simulink model "LICENTA_2024v8"  (R2018b)
settings: Solver=FixedStepDiscrete  StartTime=0.0  StopTime=Inf  RelTol=1e-3  EnableMultiTasking=on
values from neighbouring files (symbols this model uses):
  factor_conversie = (1/Rshunt)*(1/10)*(vref/4095)    (= 0.0115122972266)    [licentam18.m]
  FED = uint16(50)    [licentam18.m]
  MaxIter_1_ms_eCAP_wait = MinDetectSpeed_period/T_pos    (= 375)    [licentam18.m]
  offset_ADC = xT*4095/vref    (= 2047.5)    [licentam18.m]
  pp = 16/2    (= 8)    [licentam18.m]
  RED = uint16(50)    [licentam18.m]
  T_pos = 5*10^-4    (= 0.0005)    [licentam18.m]
  TBPRD1 = uint16(TPWM/(2*TTBCLK))    [licentam18.m]
  Tf = 0.015    [licentam18.m]
  Tf_spd = 0.01    [licentam18.m]
  TiSamplePos = T_pos    (= 0.0005)    [licentam18.m]
  Ts = Ts_crt_control    (= 3.33333333333e-05)    [licentam18.m]
  TTBCLK = 1/F    (= 5e-09)    [licentam18.m]
undefined symbols (not defined in the file or in its folder): Discrete, Down, GPTRIP1SEL, GPTRIP2SEL, radians, Time, TZ1, TZ2, Up
libraries: tiiqmathlib x25, c2802xlib x6, c2837xDlib x6, c280xlib x4, simulink x3, ctrlSharedLib x2, c2000lib x1, c28xdmclib x1
(part 1 of 2)
settings Model: ExtModeTrigDuration=8  Creator=mocan  LastModifiedBy=antic
settings SolverCC: AutoInsertRateTranBlk=on
settings OptimizationCC: DefaultUnderspecifiedDataType=single  EnhancedBackFolding=on  PassReuseOutputArgsAs=Individual arguments  MaxStackSize=512  OptimizeBlockOrder=speed  DifferentSizesBufferReuse=on  OptimizationCustomize=off
settings DebuggingCC: ParameterPrecisionLossMsg=none  ParameterTunabilityLossMsg=error
settings HardwareCC: ProdBitPerChar=16  ProdBitPerInt=16  ProdBitPerPointer=32  ProdBitPerSizeT=32  ProdBitPerPtrDiffT=32  ProdLargestAtomicInteger=Integer  ProdLargestAtomicFloat=None  ProdWordSize=16  ProdLongLongMode=on  ProdHWDeviceType=Texas Instruments->C2000
settings SFSimCC: MATLABDynamicMemAlloc=off
settings RTWCC: SystemTargetFile=ert.tlc  HardwareBoard=TI Delfino F28379D LaunchPad  TemplateMakefile=ert_default_tmf  GenerateReport=on  Toolchain=Texas Instruments Code Composer Studio (C2000)  IncludeHyperlinkInReport=on  LaunchReport=on  GenerateTraceInfo=on  GenerateTraceReport=on  GenerateTraceReportSl=on  GenerateTraceReportSf=on  GenerateTraceReportEml=on
settings CodeAppCC: ForceParamTrailComments=on  IgnoreCustomStorageClasses=off  OperatorAnnotations=on  SimulinkDataObjDesc=on  SFDataObjDesc=on  InsertBlockDesc=on
settings ERTTargetCC: CodeReplacementLibrary=TI C28x

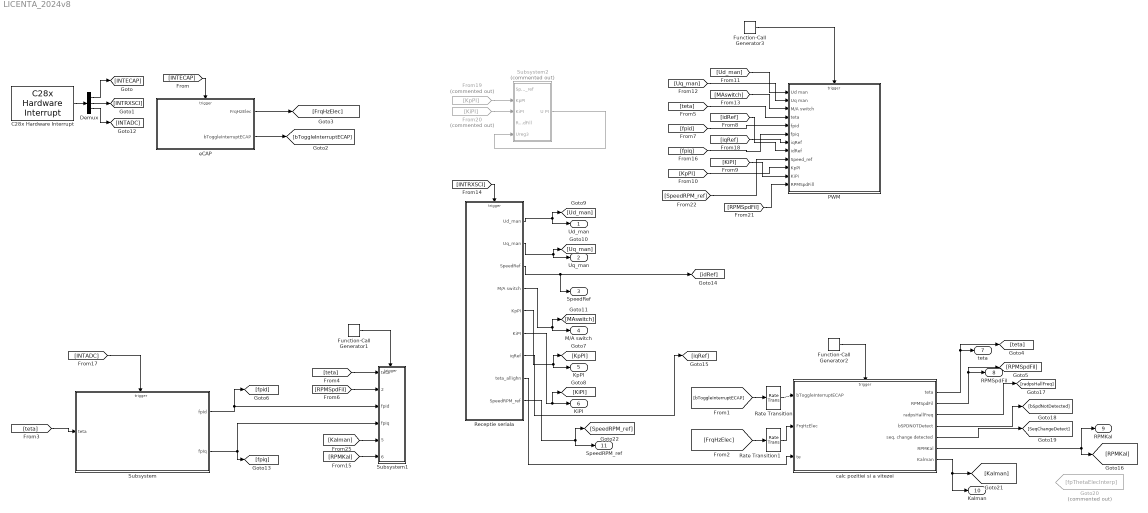
== system LICENTA_2024v8 ==
  C28x Hardware Interrupt : c2000lib/Scheduling/C28x Hardware Interrupt  irqnumbers=[4,9,1]  pienumbers=[1,1,1]  irqpriorities=[1, 1, 1]  irqpreempts=[0 0 0]  showinput=off  dspchiptype=C280X
      settings: SourceProductBaseCode=TIC2000
  Demux : Demux  Outputs=3
  From19 : From  Commented=on  GotoTag=KpPI
  From20 : From  Commented=on  GotoTag=KiPI
  Function-Call Generator1 : simulink/Ports & Subsystems/Function-Call Generator  sample_time=0.03  numberOfIterations=1
  Function-Call Generator2 : simulink/Ports & Subsystems/Function-Call Generator  sample_time=T_pos  numberOfIterations=1
  Function-Call Generator3 : simulink/Ports & Subsystems/Function-Call Generator  sample_time=Ts_crt_control  numberOfIterations=1
  Goto20 : Goto  Commented=on  GotoTag=fpThetaElecInterp
  PWM : Subsystem
  Rate Transition : RateTransition  Integrity=off  OutPortSampleTime=T_pos
  Rate Transition1 : RateTransition  Integrity=off  OutPortSampleTime=T_pos
  "Receptie seriala " : Subsystem
  Subsystem : Subsystem
  Subsystem1 : Subsystem
  Subsystem2 : Subsystem  Commented=on
  calc pozitiei si a vitezei : Subsystem
  eCAP : Subsystem
  Ud_man : Outport  VectorParamsAs1DForOutWhenUnconnected=on
  Uq_man : Outport  Port=2  VectorParamsAs1DForOutWhenUnconnected=on
  SpeedRef : Outport  Port=3  VectorParamsAs1DForOutWhenUnconnected=on
  M/A switch : Outport  Port=4  VectorParamsAs1DForOutWhenUnconnected=on
  KpPI : Outport  Port=5  VectorParamsAs1DForOutWhenUnconnected=on
  KiPI : Outport  Port=6  VectorParamsAs1DForOutWhenUnconnected=on
  teta : Outport  Port=7  VectorParamsAs1DForOutWhenUnconnected=on
  RPMSpdFil : Outport  Port=8  VectorParamsAs1DForOutWhenUnconnected=on
  RPMKal : Outport  Port=9  VectorParamsAs1DForOutWhenUnconnected=on
  Kalman : Outport  Port=10
  SpeedRPM_ref : Outport  Port=11  VectorParamsAs1DForOutWhenUnconnected=on
  wires:
  Rate Transition1/1 -> calc pozitiei si a vitezei/2(FrqHzElec)
  [FrqHzElec] -> Rate Transition1/1
  Rate Transition/1 -> calc pozitiei si a vitezei/1(bToggleInterruptECAP)
  [bToggleInterruptECAP] -> Rate Transition/1
  [INTECAP] -> eCAP/Trigger
  eCAP/1(FrqHzElec) -> [FrqHzElec]
  eCAP/2(bToggleInterruptECAP) -> [bToggleInterruptECAP]
  Demux/2 -> [INTRXSCI]
  Demux/1 -> [INTECAP]
  Function-Call Generator2/1 -> calc pozitiei si a vitezei/Trigger
  calc pozitiei si a vitezei/2(RPMSpdFil) -> [RPMSpdFil], RPMSpdFil/1
  Function-Call Generator1/1 -> Subsystem1/Trigger
  calc pozitiei si a vitezei/1(teta) -> [teta], teta/1
  [INTRXSCI] -> "Receptie seriala "/Trigger
  C28x Hardware Interrupt/1 -> Demux/1
  "Receptie seriala "/1(Ud_man) -> Ud_man/1, [Ud_man]
  "Receptie seriala "/2(Uq_man) -> Uq_man/1, [Uq_man]
  "Receptie seriala "/4(M/A switch) -> M/A switch/1, [MAswitch]
  "Receptie seriala "/5(KpPI) -> KpPI/1, [KpPI]
  "Receptie seriala "/6(KiPI) -> [KiPI], KiPI/1
  Function-Call Generator3/1 -> PWM/Trigger
  Demux/3 -> [INTADC]
  [INTADC] -> Subsystem/Trigger
  [teta] -> Subsystem/1(teta)
  Subsystem/1(fpId) -> [fpid], Subsystem1/3(fpId)
  Subsystem/2(fpIq) -> Subsystem1/4(fpIq), [fpiq]
  "Receptie seriala "/7(iqRef) -> [iqRef]
  "Receptie seriala "/3(SpeedRef) -> SpeedRef/1, [idRef]
  [Ud_man] -> PWM/1(Ud man)
  [Uq_man] -> PWM/2("Uq man ")
  [MAswitch] -> PWM/3(M/A switch)
  [teta] -> PWM/4("teta ")
  [idRef] -> PWM/8(idRef)
  [fpid] -> PWM/5(fpid)
  [fpiq] -> PWM/6(fpiq)
  [iqRef] -> PWM/7("iqRef ")
  [KiPI] -> PWM/11("KiPi ")
  [KpPI] -> PWM/10(KpPI)
  [RPMSpdFil] -> Subsystem1/2("RPMSpdFil ")
  "Receptie seriala "/8(teta_allighn) -> calc pozitiei si a vitezei/3(te)
  calc pozitiei si a vitezei/3(radpsHallFreq) -> [radpsHallFreq]
  calc pozitiei si a vitezei/4("bSPDNOTDetect ") -> [bSpdNotDetected]
  calc pozitiei si a vitezei/5("seq. change detected ") -> [SeqChangeDetect]
  [teta] -> Subsystem1/1("teta ")
  [RPMKal] -> Subsystem1/6(RPMKal)
  calc pozitiei si a vitezei/6(RPMKal) -> RPMKal/1, [RPMKal]
  calc pozitiei si a vitezei/7(Kalman) -> Kalman/1, [Kalman]
  [Kalman] -> Subsystem1/5(Kalman)
  "Receptie seriala "/9("SpeedRPM_ref ") -> [SpeedRPM_ref], SpeedRPM_ref/1
  From20/1 -> Subsystem2/3(KiPI)
  Subsystem2/1("U PI ") -> Subsystem2/5(Ureg3)
  From19/1 -> Subsystem2/2(KpPI)
  [SpeedRPM_ref] -> PWM/9(Speed_ref)
  [RPMSpdFil] -> PWM/12(RPMSpdFill)

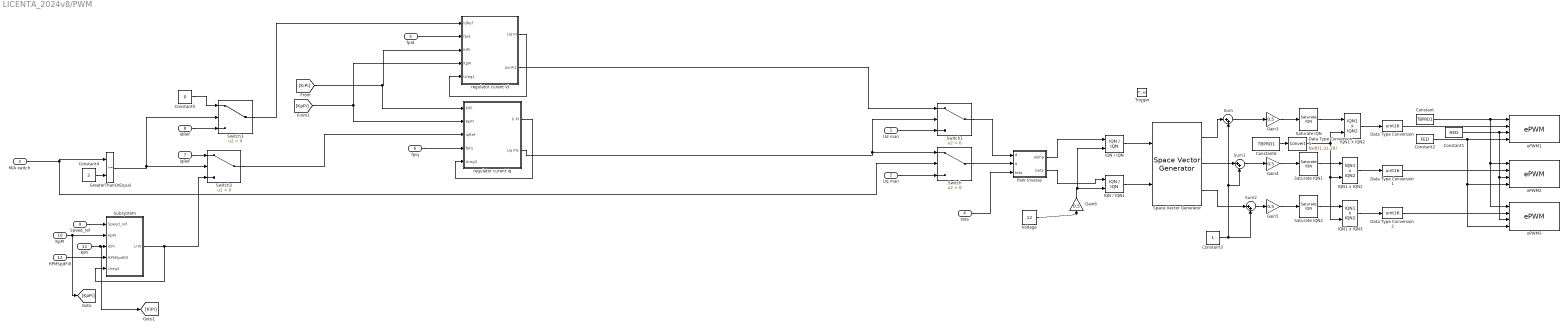
== system LICENTA_2024v8/PWM ==
  Ud man : Inport
  "Uq man " : Inport  Port=2
  M/A switch : Inport  Port=3
  "teta " : Inport  Port=4
  fpid : Inport  Port=5
  fpiq : Inport  Port=6
  "iqRef " : Inport  Port=7
  idRef : Inport  Port=8
  Speed_ref : Inport  Port=9
  KpPI : Inport  Port=10
  "KiPi " : Inport  Port=11
  RPMSpdFill : Inport  Port=12
  Trigger : TriggerPort  TriggerType=function-call  VariantControl=Variant  PortDimensions=1
  Constant : Constant  Value=TBPRD1
  Constant1 : Constant  Value=RED
  Constant2 : Constant  Value=FED
  Constant3 : Constant  OutDataTypeStr=fixdt(1,32,24)
  Constant4 : Constant  Value=2
  Constant5 : Constant  Value=0
  Constant6 : Constant  Value=TBPRD1
  Data Type Conversion : DataTypeConversion  OutDataTypeStr=uint16
  Data Type Conversion1 : DataTypeConversion  OutDataTypeStr=uint16
  Data Type Conversion2 : DataTypeConversion  OutDataTypeStr=uint16
  Data Type Conversion5 : DataTypeConversion  OutDataTypeStr=fixdt(1,32,18)
  Gain{3..6} (4 alike) : Gain  Gain=0.5  OutDataTypeStr=Inherit: Same as input
  GreaterThanOrEqual : RelationalOperator  OutDataTypeStr=boolean  RndMeth=Simplest
  IQN / IQN : tiiqmathlib/IQN // IQN
      settings: SourceProductName=Embedded Coder Support Package for Texas Instruments C2000 Processors  SourceProductBaseCode=TIC2000
  IQN / IQN1 : tiiqmathlib/IQN // IQN
      settings: SourceProductName=Embedded Coder Support Package for Texas Instruments C2000 Processors  SourceProductBaseCode=TIC2000
  IQN1 x IQN1 : tiiqmathlib/IQN1 x IQN2  Q=10
      settings: SourceProductName=Embedded Coder Support Package for Texas Instruments C2000 Processors  SourceProductBaseCode=TIC2000
  IQN1 x IQN2 : tiiqmathlib/IQN1 x IQN2  Q=10
      settings: SourceProductName=Embedded Coder Support Package for Texas Instruments C2000 Processors  SourceProductBaseCode=TIC2000
  IQN1 x IQN3 : tiiqmathlib/IQN1 x IQN2  Q=10
      settings: SourceProductName=Embedded Coder Support Package for Texas Instruments C2000 Processors  SourceProductBaseCode=TIC2000
  Park Inverse : Subsystem
  Saturate IQN : tiiqmathlib/Saturate IQN  pos=0.95  neg=0.05
      settings: SourceProductName=Embedded Coder Support Package for Texas Instruments C2000 Processors  SourceProductBaseCode=TIC2000
  Saturate IQN1 : tiiqmathlib/Saturate IQN  pos=0.95  neg=0.05
      settings: SourceProductName=Embedded Coder Support Package for Texas Instruments C2000 Processors  SourceProductBaseCode=TIC2000
  Saturate IQN2 : tiiqmathlib/Saturate IQN  pos=0.95  neg=0.05
      settings: SourceProductName=Embedded Coder Support Package for Texas Instruments C2000 Processors  SourceProductBaseCode=TIC2000
  Space Vector Generator : c28xdmclib/Space Vector Generator
      settings: SourceProductName=Embedded Coder Support Package for Texas Instruments C2000 Processors  SourceProductBaseCode=TIC2000
  Subsystem : Subsystem
  Sum : Sum  Inputs=|++
  Sum1 : Sum  Inputs=|++
  Sum2 : Sum  Inputs=|++
  Switch{,1..3} (4 alike) : Switch  Criteria=u2 > Threshold
  "Voltage " : Constant  Value=12  OutDataTypeStr=fixdt(1,32,20)
  ePWM1 : c2802xlib/ePWM  useModule=ePWM1  ePWMxLINKTBPRD=Not Linked  periodUnits=Clock cycles  timerSource=Input port  timerPeriod_clk=TBPRD1+1  timerPeriod_sec=0.0001  tbshadow=Counter equals to zero  countingMode=Up-Down  phaseActiveEnable=Disable  phaseDirection=Count up after sync  phaseActive=0  synchronizationEnable=off  dcaevt1Sync=off  dcbevt1Sync=off  synchronizationOption=Counter equals to zero (CTR=Zero)  clockPrescale=1  HSclockPrescale=1  enswap=off  ePWMxAStatus=on  ePWMxAactionLogic1=Do nothing  ePWMxAactionLogic2=Do nothing  ePWMxAactionLogic3=Clear  ePWMxAactionLogic4=Set  ePWMxAactionLogic5=Do nothing  ePWMxAactionLogic6=Do nothing  ePWMxALoadMode=Load on counter equals to zero (CTR=Zero)  ePWMxACSFenable=off  ePWMxACSFvalue=Forcing disable  ePWMxASFreload=Zero  ePWMxBStatus=off  ePWMxBactionLogic1=Set  ePWMxBactionLogic2=Clear  ePWMxBactionLogic3=Do nothing  ePWMxBactionLogic4=Do nothing  ePWMxBactionLogic5=Clear  ePWMxBactionLogic6=Set  ePWMxBLoadMode=Load on counter equals to zero (CTR=Zero)  ePWMxBCSFenable=off  ePWMxBCSFvalue=Forcing disable  ePWMxBSFreload=Zero  ePWNxBOutWay=off  ePWMxLINKCMPA=Not Linked  CMPAUnits=Clock cycles  CMPASource=Input port  CMPAValue_per=50  CMPAValue_clk=0  enCMPAshadow=Counter equals to zero  ePWMxLINKCMPB=Not Linked  CMPBUnits=Clock cycles  CMPBSource=Specify via dialog  CMPBValue_per=50  CMPBValue_clk=0  enCMPBshadow=Counter equals to zero  ePWMxLINKCMPC=Not Linked  CMPCUnits=Clock cycles  CMPCSource=Specify via dialog  CMPCValue_per=50  CMPCValue_clk=32000  enCMPCshadow=Counter equals to zero  ePWMxLINKCMPD=Not Linked  CMPDUnits=Clock cycles  CMPDSource=Specify via dialog  CMPDValue_per=50  CMPDValue_clk=32000  enCMPDshadow=Counter equals to zero  enableDBePWMxA=on  enableDBePWMxB=on  enhalfcycle=off  DBpolarity=Active high complementary (AHC)  DBedgeDelay=Positive  DBSource_ePWMxA=ePWMxA  DBSource_ePWMxB=ePWMxA  DBperiodSource=Input port  REDperiod=0  FEDperiod=0  adcstartModuleA=on  adcrequestEventA=First event  adcstartEventA=Digital Compare Module A Event 1 start of conversion (DCAEVT1.soc)  adcstartEventA_type2=Counter equals to period (CTR=PRD)  adcstartModuleB=off  adcrequestEventB=First event  adcstartEventB=Counter equals to zero (CTR=Zero)  adcstartEventB_type2=Counter equals to zero (CTR=Zero)  intEn=off  intPrd=First event  intSel=Counter equals to zero (CTR=Zero)  intSel_type2=Counter equals to zero (CTR=Zero)  hrpe=off  enHRPWM=off  HRPWM_LoadMode=Counter equals to period (CTR=PRD)  HRPWM_CTLMode=Duty or Period control mode  HRPWM_EDGMode=Both edge  hrpeb=off  enHRPWMB=off  HRPWM_LoadModeB=Counter equals to zero (CTR=ZERO)  HRPWM_CTLModeB=Duty or Period control mode  HRPWM_EDGModeB=Both edge  enSFO=on  enautoconv=on  chopperEnable=off  chopperFrequency=1  chopperFirstwidth=1  chopperDuty=12.5%  tripZonesource=Specify via dialog  tzselOSHT1=off  tzselOSHT2=off  tzselOSHT3=off  tzselOSHDCAEV1=off  tzselOSHDCBEV1=off  tzselCBC1=off  tzselCBC2=off  tzselCBC3=off  tzselCBCDCAEV2=off  tzselCBCDCBEV2=off  tzselOSHT4=off  tzselOSHT5=off  tzselOSHT6=off  tzselCBC4=off  tzselCBC5=off  tzselCBC6=off  enTzOstIntr=off  enTzCbcIntr=off  enTzDCAEVT1Intr=off  enTzDCAEVT2Intr=off  enTzDCBEVT1Intr=off  enTzDCBEVT2Intr=off  ePWMxAforced=No action  ePWMxBforced=No action  DCAEVT1forced=No action  DCBEVT1forced=No action  DCAEVT2forced=No action  DCBEVT2forced=No action  dcah=Trip Zone 1 input (TZ1)  dcal=Trip Zone 2 input (TZ2)  dcbh=Trip Zone 1 input (TZ1)  dcbl=Trip Zone 2 input (TZ2)  dcah_type2=GPTRIP1SEL/(TZ1)  dcal_type2=GPTRIP2SEL/(TZ2)  dcbh_type2=GPTRIP1SEL/(TZ1)  dcbl_type2=GPTRIP2SEL/(TZ2)  gendcaevt1=Event disabled  gendcaevt2=Event disabled  gendcbevt1=Event disabled  gendcbevt2=Event disabled  dcaevt1src=DCAEVT1 with sync  dcaevt2src=DCAEVT2 with sync  dcbevt1src=DCBEVT1 with sync  dcbevt2src=DCBEVT2 with sync  pulsesel=Counter equals to zero (CTR=Zero)  blankinv=off  blankoffset=0  blankwidth=0  evsrcsel=Filtered version of DCAEVT1 (DCAEVT1FILT)  encape=off  PwmType=C2000_Type4
      settings: SourceProductName=Embedded Coder Support Package for Texas Instruments C2000 Processors
  ePWM2 : c2802xlib/ePWM  useModule=ePWM2  ePWMxLINKTBPRD=Not Linked  periodUnits=Clock cycles  timerSource=Input port  timerPeriod_clk=TBPRD1+1  timerPeriod_sec=0.0001  tbshadow=Counter equals to zero  countingMode=Up-Down  phaseActiveEnable=Disable  phaseDirection=Count up after sync  phaseActive=0  synchronizationEnable=off  dcaevt1Sync=off  dcbevt1Sync=off  synchronizationOption=Counter equals to zero (CTR=Zero)  clockPrescale=1  HSclockPrescale=1  enswap=off  ePWMxAStatus=on  ePWMxAactionLogic1=Do nothing  ePWMxAactionLogic2=Do nothing  ePWMxAactionLogic3=Clear  ePWMxAactionLogic4=Set  ePWMxAactionLogic5=Do nothing  ePWMxAactionLogic6=Do nothing  ePWMxALoadMode=Load on counter equals to zero (CTR=Zero)  ePWMxACSFenable=off  ePWMxACSFvalue=Forcing disable  ePWMxASFreload=Zero  ePWMxBStatus=off  ePWMxBactionLogic1=Set  ePWMxBactionLogic2=Clear  ePWMxBactionLogic3=Do nothing  ePWMxBactionLogic4=Do nothing  ePWMxBactionLogic5=Clear  ePWMxBactionLogic6=Set  ePWMxBLoadMode=Load on counter equals to zero (CTR=Zero)  ePWMxBCSFenable=off  ePWMxBCSFvalue=Forcing disable  ePWMxBSFreload=Zero  ePWNxBOutWay=off  ePWMxLINKCMPA=Not Linked  CMPAUnits=Clock cycles  CMPASource=Input port  CMPAValue_per=50  CMPAValue_clk=0  enCMPAshadow=Counter equals to zero  ePWMxLINKCMPB=Not Linked  CMPBUnits=Clock cycles  CMPBSource=Specify via dialog  CMPBValue_per=50  CMPBValue_clk=0  enCMPBshadow=Counter equals to zero  ePWMxLINKCMPC=Not Linked  CMPCUnits=Clock cycles  CMPCSource=Specify via dialog  CMPCValue_per=50  CMPCValue_clk=32000  enCMPCshadow=Counter equals to zero  ePWMxLINKCMPD=Not Linked  CMPDUnits=Clock cycles  CMPDSource=Specify via dialog  CMPDValue_per=50  CMPDValue_clk=32000  enCMPDshadow=Counter equals to zero  enableDBePWMxA=on  enableDBePWMxB=on  enhalfcycle=off  DBpolarity=Active high complementary (AHC)  DBedgeDelay=Positive  DBSource_ePWMxA=ePWMxA  DBSource_ePWMxB=ePWMxA  DBperiodSource=Input port  REDperiod=0  FEDperiod=0  adcstartModuleA=on  adcrequestEventA=First event  adcstartEventA=Digital Compare Module A Event 1 start of conversion (DCAEVT1.soc)  adcstartEventA_type2=Counter equals to period (CTR=PRD)  adcstartModuleB=off  adcrequestEventB=First event  adcstartEventB=Counter equals to zero (CTR=Zero)  adcstartEventB_type2=Counter equals to zero (CTR=Zero)  intEn=off  intPrd=First event  intSel=Counter equals to zero (CTR=Zero)  intSel_type2=Counter equals to zero (CTR=Zero)  hrpe=off  enHRPWM=off  HRPWM_LoadMode=Counter equals to period (CTR=PRD)  HRPWM_CTLMode=Duty or Period control mode  HRPWM_EDGMode=Both edge  hrpeb=off  enHRPWMB=off  HRPWM_LoadModeB=Counter equals to zero (CTR=ZERO)  HRPWM_CTLModeB=Duty or Period control mode  HRPWM_EDGModeB=Both edge  enSFO=on  enautoconv=on  chopperEnable=off  chopperFrequency=1  chopperFirstwidth=1  chopperDuty=12.5%  tripZonesource=Specify via dialog  tzselOSHT1=off  tzselOSHT2=off  tzselOSHT3=off  tzselOSHDCAEV1=off  tzselOSHDCBEV1=off  tzselCBC1=off  tzselCBC2=off  tzselCBC3=off  tzselCBCDCAEV2=off  tzselCBCDCBEV2=off  tzselOSHT4=off  tzselOSHT5=off  tzselOSHT6=off  tzselCBC4=off  tzselCBC5=off  tzselCBC6=off  enTzOstIntr=off  enTzCbcIntr=off  enTzDCAEVT1Intr=off  enTzDCAEVT2Intr=off  enTzDCBEVT1Intr=off  enTzDCBEVT2Intr=off  ePWMxAforced=No action  ePWMxBforced=No action  DCAEVT1forced=No action  DCBEVT1forced=No action  DCAEVT2forced=No action  DCBEVT2forced=No action  dcah=Trip Zone 1 input (TZ1)  dcal=Trip Zone 2 input (TZ2)  dcbh=Trip Zone 1 input (TZ1)  dcbl=Trip Zone 2 input (TZ2)  dcah_type2=GPTRIP1SEL/(TZ1)  dcal_type2=GPTRIP2SEL/(TZ2)  dcbh_type2=GPTRIP1SEL/(TZ1)  dcbl_type2=GPTRIP2SEL/(TZ2)  gendcaevt1=Event disabled  gendcaevt2=Event disabled  gendcbevt1=Event disabled  gendcbevt2=Event disabled  dcaevt1src=DCAEVT1 with sync  dcaevt2src=DCAEVT2 with sync  dcbevt1src=DCBEVT1 with sync  dcbevt2src=DCBEVT2 with sync  pulsesel=Counter equals to zero (CTR=Zero)  blankinv=off  blankoffset=0  blankwidth=0  evsrcsel=Filtered version of DCAEVT1 (DCAEVT1FILT)  encape=off  PwmType=C2000_Type4
      settings: SourceProductName=Embedded Coder Support Package for Texas Instruments C2000 Processors
  ePWM3 : c2802xlib/ePWM  useModule=ePWM3  ePWMxLINKTBPRD=Not Linked  periodUnits=Clock cycles  timerSource=Input port  timerPeriod_clk=TBPRD1+1  timerPeriod_sec=0.0001  tbshadow=Counter equals to zero  countingMode=Up-Down  phaseActiveEnable=Disable  phaseDirection=Count up after sync  phaseActive=0  synchronizationEnable=off  dcaevt1Sync=off  dcbevt1Sync=off  synchronizationOption=Counter equals to zero (CTR=Zero)  clockPrescale=1  HSclockPrescale=1  enswap=off  ePWMxAStatus=on  ePWMxAactionLogic1=Do nothing  ePWMxAactionLogic2=Do nothing  ePWMxAactionLogic3=Clear  ePWMxAactionLogic4=Set  ePWMxAactionLogic5=Do nothing  ePWMxAactionLogic6=Do nothing  ePWMxALoadMode=Load on counter equals to zero (CTR=Zero)  ePWMxACSFenable=off  ePWMxACSFvalue=Forcing disable  ePWMxASFreload=Zero  ePWMxBStatus=off  ePWMxBactionLogic1=Set  ePWMxBactionLogic2=Clear  ePWMxBactionLogic3=Do nothing  ePWMxBactionLogic4=Do nothing  ePWMxBactionLogic5=Clear  ePWMxBactionLogic6=Set  ePWMxBLoadMode=Load on counter equals to zero (CTR=Zero)  ePWMxBCSFenable=off  ePWMxBCSFvalue=Forcing disable  ePWMxBSFreload=Zero  ePWNxBOutWay=off  ePWMxLINKCMPA=Not Linked  CMPAUnits=Clock cycles  CMPASource=Input port  CMPAValue_per=50  CMPAValue_clk=0  enCMPAshadow=Counter equals to zero  ePWMxLINKCMPB=Not Linked  CMPBUnits=Clock cycles  CMPBSource=Specify via dialog  CMPBValue_per=50  CMPBValue_clk=0  enCMPBshadow=Counter equals to zero  ePWMxLINKCMPC=Not Linked  CMPCUnits=Clock cycles  CMPCSource=Specify via dialog  CMPCValue_per=50  CMPCValue_clk=32000  enCMPCshadow=Counter equals to zero  ePWMxLINKCMPD=Not Linked  CMPDUnits=Clock cycles  CMPDSource=Specify via dialog  CMPDValue_per=50  CMPDValue_clk=32000  enCMPDshadow=Counter equals to zero  enableDBePWMxA=on  enableDBePWMxB=on  enhalfcycle=off  DBpolarity=Active high complementary (AHC)  DBedgeDelay=Positive  DBSource_ePWMxA=ePWMxA  DBSource_ePWMxB=ePWMxA  DBperiodSource=Input port  REDperiod=0  FEDperiod=0  adcstartModuleA=on  adcrequestEventA=First event  adcstartEventA=Digital Compare Module A Event 1 start of conversion (DCAEVT1.soc)  adcstartEventA_type2=Counter equals to period (CTR=PRD)  adcstartModuleB=off  adcrequestEventB=First event  adcstartEventB=Counter equals to zero (CTR=Zero)  adcstartEventB_type2=Counter equals to zero (CTR=Zero)  intEn=off  intPrd=First event  intSel=Counter equals to zero (CTR=Zero)  intSel_type2=Counter equals to zero (CTR=Zero)  hrpe=off  enHRPWM=off  HRPWM_LoadMode=Counter equals to period (CTR=PRD)  HRPWM_CTLMode=Duty or Period control mode  HRPWM_EDGMode=Both edge  hrpeb=off  enHRPWMB=off  HRPWM_LoadModeB=Counter equals to zero (CTR=ZERO)  HRPWM_CTLModeB=Duty or Period control mode  HRPWM_EDGModeB=Both edge  enSFO=on  enautoconv=on  chopperEnable=off  chopperFrequency=1  chopperFirstwidth=1  chopperDuty=12.5%  tripZonesource=Specify via dialog  tzselOSHT1=off  tzselOSHT2=off  tzselOSHT3=off  tzselOSHDCAEV1=off  tzselOSHDCBEV1=off  tzselCBC1=off  tzselCBC2=off  tzselCBC3=off  tzselCBCDCAEV2=off  tzselCBCDCBEV2=off  tzselOSHT4=off  tzselOSHT5=off  tzselOSHT6=off  tzselCBC4=off  tzselCBC5=off  tzselCBC6=off  enTzOstIntr=off  enTzCbcIntr=off  enTzDCAEVT1Intr=off  enTzDCAEVT2Intr=off  enTzDCBEVT1Intr=off  enTzDCBEVT2Intr=off  ePWMxAforced=No action  ePWMxBforced=No action  DCAEVT1forced=No action  DCBEVT1forced=No action  DCAEVT2forced=No action  DCBEVT2forced=No action  dcah=Trip Zone 1 input (TZ1)  dcal=Trip Zone 2 input (TZ2)  dcbh=Trip Zone 1 input (TZ1)  dcbl=Trip Zone 2 input (TZ2)  dcah_type2=GPTRIP1SEL/(TZ1)  dcal_type2=GPTRIP2SEL/(TZ2)  dcbh_type2=GPTRIP1SEL/(TZ1)  dcbl_type2=GPTRIP2SEL/(TZ2)  gendcaevt1=Event disabled  gendcaevt2=Event disabled  gendcbevt1=Event disabled  gendcbevt2=Event disabled  dcaevt1src=DCAEVT1 with sync  dcaevt2src=DCAEVT2 with sync  dcbevt1src=DCBEVT1 with sync  dcbevt2src=DCBEVT2 with sync  pulsesel=Counter equals to zero (CTR=Zero)  blankinv=off  blankoffset=0  blankwidth=0  evsrcsel=Filtered version of DCAEVT1 (DCAEVT1FILT)  encape=off  PwmType=C2000_Type4
      settings: SourceProductName=Embedded Coder Support Package for Texas Instruments C2000 Processors
  regulator curent id : Subsystem
  regulator curent iq : Subsystem
  wires:
  Constant/1 -> ePWM3/1, ePWM2/1, ePWM1/1
  Constant1/1 -> ePWM3/3, ePWM2/3, ePWM1/3
  Constant2/1 -> ePWM3/4, ePWM2/4, ePWM1/4
  Data Type Conversion/1 -> ePWM1/2
  Data Type Conversion1/1 -> ePWM2/2
  Data Type Conversion2/1 -> ePWM3/2
  IQN1 x IQN2/1 -> Data Type Conversion/1
  IQN1 x IQN1/1 -> Data Type Conversion1/1
  IQN1 x IQN3/1 -> Data Type Conversion2/1
  Saturate IQN/1 -> IQN1 x IQN2/1
  Saturate IQN1/1 -> IQN1 x IQN1/1
  Gain5/1 -> Saturate IQN2/1
  Gain4/1 -> Saturate IQN1/1
  Gain3/1 -> Saturate IQN/1
  Sum/1 -> Gain3/1
  Sum1/1 -> Gain4/1
  Sum2/1 -> Gain5/1
  Space Vector Generator/1 -> Sum/1
  Space Vector Generator/2 -> Sum1/1
  Space Vector Generator/3 -> Sum2/1
  Park Inverse/1(alpha) -> IQN / IQN/1
  Park Inverse/2(beta) -> IQN / IQN1/1
  Constant3/1 -> Sum1/2, Sum/2, Sum2/2
  "Voltage "/1 -> Gain6/1
  Gain6/1 -> IQN / IQN1/2, IQN / IQN/2
  M/A switch/1 -> GreaterThanOrEqual/1, Switch/2
  "Uq man "/1 -> Switch/3
  "teta "/1 -> Park Inverse/3(teta)
  IQN / IQN/1 -> Space Vector Generator/1
  IQN / IQN1/1 -> Space Vector Generator/2
  Saturate IQN2/1 -> IQN1 x IQN3/1
  Switch/1 -> Park Inverse/2(q)
  Constant6/1 -> Data Type Conversion5/1
  Data Type Conversion5/1 -> IQN1 x IQN2/2, IQN1 x IQN3/2, IQN1 x IQN1/2
  Switch1/1 -> Park Inverse/1(d)
  regulator curent id/2(Ud PI1) -> Switch1/1
  Ud man/1 -> Switch1/3
  regulator curent iq/2(Uq PI1) -> Switch1/2, Switch/1
  Switch2/1 -> regulator curent iq/3(iqRef)
  fpiq/1 -> regulator curent iq/4(fpiq)
  [KiPi] -> regulator curent iq/1(KiPI), regulator curent id/3(KiPI)
  [KpPi] -> regulator curent iq/2(KpPI), regulator curent id/4(KpPI)
  regulator curent id/1(Ud PI) -> regulator curent id/5(Ureg1)
  fpid/1 -> regulator curent id/2(fpid)
  regulator curent iq/1(U PI) -> regulator curent iq/5(Ureg3)
  Constant4/1 -> GreaterThanOrEqual/2
  Constant5/1 -> Switch3/1
  GreaterThanOrEqual/1 -> Switch3/2, Switch2/2
  idRef/1 -> Switch3/3
  "iqRef "/1 -> Switch2/1
  Switch3/1 -> regulator curent id/1(idRef)
  Speed_ref/1 -> Subsystem/1(Speed_ref)
  RPMSpdFill/1 -> Subsystem/4(RPMSpdFill)
  Subsystem/1("U PI ") -> Subsystem/5(Ureg3), Switch2/3
  KpPI/1 -> [KpPi], Subsystem/2(KpPI)
  "KiPi "/1 -> [KiPi], Subsystem/3("KiPi ")

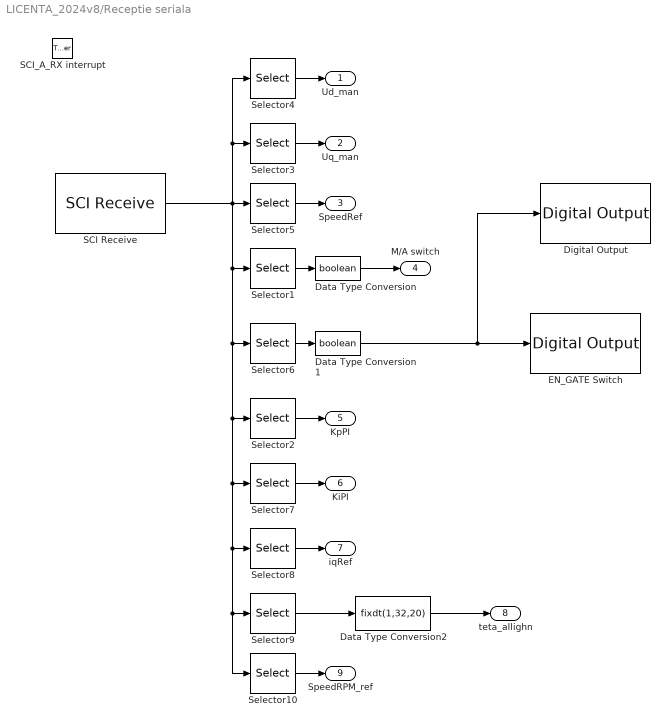
== system LICENTA_2024v8/Receptie seriala  ==
  "SCI_A_RX interrupt " : TriggerPort  TriggerType=function-call  VariantControl=(inherit)  PortDimensions=1
  Data Type Conversion : DataTypeConversion  OutDataTypeStr=boolean
  Data Type Conversion1 : DataTypeConversion  OutDataTypeStr=boolean
  Data Type Conversion2 : DataTypeConversion  OutDataTypeStr=fixdt(1,32,20)
  Digital Output : c2837xDlib/Digital Output  GPIO_Number=GPIO88~GPIO95  GPIO_Bit0=off  GPIO_BIT0_Toggle=off  GPIO_Bit1=off  GPIO_BIT1_Toggle=off  GPIO_Bit2=off  GPIO_BIT2_Toggle=off  GPIO_Bit3=off  GPIO_BIT3_Toggle=off  GPIO_Bit4=off  GPIO_BIT4_Toggle=off  GPIO_Bit5=off  GPIO_BIT5_Toggle=off  GPIO_Bit6=on  GPIO_BIT6_Toggle=off  GPIO_Bit7=off  GPIO_BIT7_Toggle=off
      settings: SourceProductName=Embedded Coder Support Package for Texas Instruments C2000 Processors  SourceProductBaseCode=TIC2000
  EN_GATE Switch : c2837xDlib/Digital Output  GPIO_Number=GPIO120~GPIO127  GPIO_Bit0=off  GPIO_BIT0_Toggle=off  GPIO_Bit1=off  GPIO_BIT1_Toggle=off  GPIO_Bit2=off  GPIO_BIT2_Toggle=off  GPIO_Bit3=off  GPIO_BIT3_Toggle=off  GPIO_Bit4=on  GPIO_BIT4_Toggle=off  GPIO_Bit5=off  GPIO_BIT5_Toggle=off  GPIO_Bit6=off  GPIO_BIT6_Toggle=off  GPIO_Bit7=off  GPIO_BIT7_Toggle=on
      settings: SourceProductName=Embedded Coder Support Package for Texas Instruments C2000 Processors  SourceProductBaseCode=TIC2000
  SCI Receive : c280xlib/SCI Receive  sciModule=A  dataHead='SS'  dataTail='EE'  dataType=single  dataDim=serial_data_length  initValue=0  errOption=Output the last received value  errValue=0  sampleTime=-1  outputStatus=off  postInterrupt=on  numFifo=4
      settings: SourceProductName=Embedded Coder Support Package for Texas Instruments C2000 Processors  SourceProductBaseCode=TIC2000
  Selector1 : Selector  InputPortWidth=serial_data_length  IndexOptions=Index vector (dialog)  Indices=[4]  OutputSizes=1
  Selector10 : Selector  InputPortWidth=serial_data_length  IndexOptions=Index vector (dialog)  Indices=[8]  OutputSizes=1
  Selector2 : Selector  InputPortWidth=serial_data_length  IndexOptions=Index vector (dialog)  Indices=[6]  OutputSizes=1
  Selector3 : Selector  InputPortWidth=serial_data_length  IndexOptions=Index vector (dialog)  Indices=[2]  OutputSizes=1
  Selector4 : Selector  InputPortWidth=serial_data_length  IndexOptions=Index vector (dialog)  Indices=[1]  OutputSizes=1
  Selector5 : Selector  InputPortWidth=serial_data_length  IndexOptions=Index vector (dialog)  Indices=[3]  OutputSizes=1
  Selector6 : Selector  InputPortWidth=serial_data_length  IndexOptions=Index vector (dialog)  Indices=[5]  OutputSizes=1
  Selector7 : Selector  InputPortWidth=serial_data_length  IndexOptions=Index vector (dialog)  Indices=[7]  OutputSizes=1
  Selector8 : Selector  InputPortWidth=serial_data_length  IndexOptions=Index vector (dialog)  Indices=[8]  OutputSizes=1
  Selector9 : Selector  InputPortWidth=serial_data_length  IndexOptions=Index vector (dialog)  Indices=[9]  OutputSizes=1
  Ud_man : Outport  VectorParamsAs1DForOutWhenUnconnected=on
  Uq_man : Outport  Port=2  VectorParamsAs1DForOutWhenUnconnected=on
  SpeedRef : Outport  Port=3  VectorParamsAs1DForOutWhenUnconnected=on
  M/A switch : Outport  Port=4  VectorParamsAs1DForOutWhenUnconnected=on
  KpPI : Outport  Port=5  VectorParamsAs1DForOutWhenUnconnected=on
  KiPI : Outport  Port=6  VectorParamsAs1DForOutWhenUnconnected=on
  iqRef : Outport  Port=7  VectorParamsAs1DForOutWhenUnconnected=on
  teta_allighn : Outport  Port=8  VectorParamsAs1DForOutWhenUnconnected=on
  "SpeedRPM_ref " : Outport  Port=9  VectorParamsAs1DForOutWhenUnconnected=on
  wires:
  SCI Receive/1 -> Selector1/1, Selector6/1, Selector2/1, Selector10/1, Selector9/1, Selector8/1, Selector7/1, Selector5/1, Selector4/1, Selector3/1
  Selector7/1 -> KiPI/1
  Selector2/1 -> KpPI/1
  Selector5/1 -> SpeedRef/1
  Selector3/1 -> Uq_man/1
  Selector4/1 -> Ud_man/1
  Selector1/1 -> Data Type Conversion/1
  Data Type Conversion/1 -> M/A switch/1
  Selector6/1 -> Data Type Conversion1/1
  Data Type Conversion1/1 -> Digital Output/1, EN_GATE Switch/1
  Selector8/1 -> iqRef/1
  Selector9/1 -> Data Type Conversion2/1
  Data Type Conversion2/1 -> teta_allighn/1
  Selector10/1 -> "SpeedRPM_ref "/1

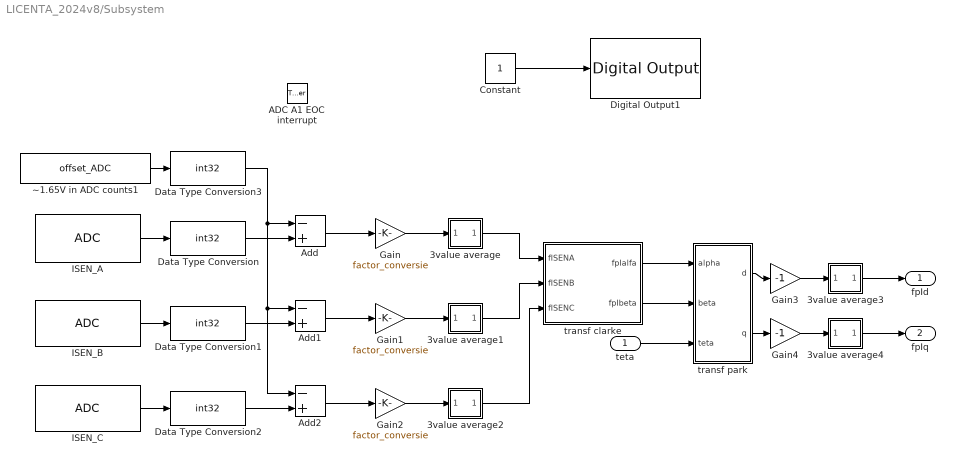
== system LICENTA_2024v8/Subsystem ==
  teta : Inport
  ADC A1 EOC interrupt : TriggerPort  TriggerType=function-call  VariantControl=Variant  PortDimensions=1
  3value average : Subsystem
  3value average1 : Subsystem
  3value average2 : Subsystem
  3value average3 : Subsystem
  3value average4 : Subsystem
  Add : Sum  Inputs=-+  OutDataTypeStr=single
  Add1 : Sum  Inputs=-+  OutDataTypeStr=single
  Add2 : Sum  Inputs=-+  OutDataTypeStr=single
  Constant : Constant
  Data Type Conversion{,1..3} (4 alike) : DataTypeConversion  OutDataTypeStr=int32  ConvertRealWorld=Stored Integer (SI)
  Digital Output1 : c2837xDlib/Digital Output  GPIO_Number=GPIO16~GPIO23  GPIO_Bit0=off  GPIO_BIT0_Toggle=off  GPIO_Bit1=off  GPIO_BIT1_Toggle=off  GPIO_Bit2=off  GPIO_BIT2_Toggle=off  GPIO_Bit3=off  GPIO_BIT3_Toggle=off  GPIO_Bit4=off  GPIO_BIT4_Toggle=off  GPIO_Bit5=off  GPIO_BIT5_Toggle=off  GPIO_Bit6=on  GPIO_BIT6_Toggle=on  GPIO_Bit7=off  GPIO_BIT7_Toggle=off
      settings: SourceProductName=Embedded Coder Support Package for Texas Instruments C2000 Processors  SourceProductBaseCode=TIC2000
  Gain : Gain  Gain=factor_conversie  OutDataTypeStr=fixdt(1,32,16)
  Gain1 : Gain  Gain=factor_conversie  OutDataTypeStr=fixdt(1,32,16)
  Gain2 : Gain  Gain=factor_conversie  OutDataTypeStr=fixdt(1,32,16)
  Gain3 : Gain  Gain=-1
  Gain4 : Gain  Gain=-1
  ISEN_A : c2802xlib/ADC  blkParamProc=C2000_Type4  ADCModule=C  samplingMode=Single sample mode  ADCResolution=12-bit (Single-ended input)  useSOC1=SOC0  useSOC2=SOC0_SOC1  SOCAcquisitionWindow=7  SOCTriggerSource=ePWM1_ADCSOCA  SOCInterruptTrigger=No ADCINT  Ts=-1  dType=uint16  postInterrupt=off  interruptSel=ADCINT2  ADCINTContinuous=on  endma=off  chdma=1  conv1=ADCINA0  conv2=ADCINA0 and ADCINB0  conv1_Type4=ADCIN2  conv2_Type4=ADCIN0 and ADCIN1
      settings: SourceProductName=Embedded Coder Support Package for Texas Instruments C2000 Processors
  ISEN_B : c2802xlib/ADC  blkParamProc=C2000_Type4  ADCModule=B  samplingMode=Single sample mode  ADCResolution=12-bit (Single-ended input)  useSOC1=SOC0  useSOC2=SOC0_SOC1  SOCAcquisitionWindow=7  SOCTriggerSource=ePWM1_ADCSOCA  SOCInterruptTrigger=No ADCINT  Ts=-1  dType=uint16  postInterrupt=off  interruptSel=ADCINT2  ADCINTContinuous=on  endma=off  chdma=1  conv1=ADCINA0  conv2=ADCINA0 and ADCINB0  conv1_Type4=ADCIN2  conv2_Type4=ADCIN0 and ADCIN1
      settings: SourceProductName=Embedded Coder Support Package for Texas Instruments C2000 Processors
  ISEN_C : c2802xlib/ADC  blkParamProc=C2000_Type4  ADCModule=A  samplingMode=Single sample mode  ADCResolution=12-bit (Single-ended input)  useSOC1=SOC0  useSOC2=SOC0_SOC1  SOCAcquisitionWindow=15  SOCTriggerSource=ePWM1_ADCSOCA  SOCInterruptTrigger=No ADCINT  Ts=-1  dType=uint16  postInterrupt=on  interruptSel=ADCINT1  ADCINTContinuous=on  endma=off  chdma=1  conv1=ADCINA0  conv2=ADCINA0 and ADCINB0  conv1_Type4=ADCIN2  conv2_Type4=ADCIN0 and ADCIN1
      settings: SourceProductName=Embedded Coder Support Package for Texas Instruments C2000 Processors
  transf clarke : Subsystem
  transf park : Subsystem
  ~1.65V in ADC counts1 : Constant  Value=offset_ADC  OutDataTypeStr=int32
  fpId : Outport
  fpIq : Outport  Port=2
  wires:
  3value average2/1(out) -> transf clarke/3(fISENC)
  3value average1/1(out) -> transf clarke/2(fISENB)
  3value average/1(out) -> transf clarke/1(fISENA)
  transf clarke/2(fpIbeta) -> transf park/2(beta)
  transf clarke/1(fpIalfa) -> transf park/1(alpha)
  teta/1 -> transf park/3("teta ")
  Data Type Conversion3/1 -> Add/1, Add1/1, Add2/1
  ISEN_B/1 -> Data Type Conversion1/1
  ISEN_C/1 -> Data Type Conversion2/1
  Data Type Conversion2/1 -> Add2/2
  Data Type Conversion1/1 -> Add1/2
  ~1.65V in ADC counts1/1 -> Data Type Conversion3/1
  Data Type Conversion/1 -> Add/2
  ISEN_A/1 -> Data Type Conversion/1
  Add/1 -> Gain/1
  Gain/1 -> 3value average/1(in)
  Add1/1 -> Gain1/1
  Gain1/1 -> 3value average1/1(in)
  Add2/1 -> Gain2/1
  Gain2/1 -> 3value average2/1(in)
  Constant/1 -> Digital Output1/1
  transf park/1(d) -> Gain3/1
  transf park/2(q) -> Gain4/1
  Gain3/1 -> 3value average3/1(in)
  Gain4/1 -> 3value average4/1(in)
  3value average3/1(out) -> fpId/1
  3value average4/1(out) -> fpIq/1

== system LICENTA_2024v8/Subsystem1 ==
  "teta " : Inport
  "RPMSpdFil " : Inport  Port=2
  fpId : Inport  Port=3
  fpIq : Inport  Port=4
  Kalman : Inport  Port=5
  RPMKal : Inport  Port=6
  Trigger : TriggerPort  TriggerType=function-call  VariantControl=(inherit)  SampleTime=-1  PortDimensions=1
  Data Type Conversion{1..6} (6 alike) : DataTypeConversion  OutDataTypeStr=single
  Mux : Mux  Inputs=6
  SCI Transmit : c280xlib/SCI Transmit  sciModule=A  dataHead='S'  dataTail='E'  postInterrupt=off  numFifo=1
      settings: SourceProductName=Embedded Coder Support Package for Texas Instruments C2000 Processors
  wires:
  "teta "/1 -> Data Type Conversion1/1
  "RPMSpdFil "/1 -> Data Type Conversion2/1
  Data Type Conversion2/1 -> Mux/2
  Mux/1 -> SCI Transmit/1
  Data Type Conversion1/1 -> Mux/1
  fpId/1 -> Data Type Conversion3/1
  Data Type Conversion3/1 -> Mux/3
  Data Type Conversion4/1 -> Mux/4
  Data Type Conversion6/1 -> Mux/6
  RPMKal/1 -> Data Type Conversion6/1
  Data Type Conversion5/1 -> Mux/5
  fpIq/1 -> Data Type Conversion4/1
  Kalman/1 -> Data Type Conversion5/1

== system LICENTA_2024v8/Subsystem2 ==
  Speed_ref : Inport
  KpPI : Inport  Port=2
  KiPI : Inport  Port=3
  RPMSpdFill : Inport  Port=4
  Ureg3 : Inport  Port=5
  Constant : Constant  Value=Ts
  Product : Product
  Product1 : Product
  Product2 : Product
  Sum : Sum  Inputs=|++
  Sum1 : Sum  Inputs=|+-
  Sum2 : Sum  Inputs=|+-+
  Unit Delay : UnitDelay  SampleTime=-1
  Unit Delay1 : UnitDelay  SampleTime=-1
  "U PI " : Outport
  wires:
  Speed_ref/1 -> Sum1/1
  KiPI/1 -> Product/1
  Constant/1 -> Product/2
  Product/1 -> Sum/1
  KpPI/1 -> Sum/2, Product2/1
  Sum/1 -> Product1/1
  Sum1/1 -> Unit Delay/1, Product1/2
  Unit Delay/1 -> Product2/2
  RPMSpdFill/1 -> Sum1/2
  Ureg3/1 -> Unit Delay1/1
  Sum2/1 -> "U PI "/1
  Unit Delay1/1 -> Sum2/3
  Product2/1 -> Sum2/2
  Product1/1 -> Sum2/1

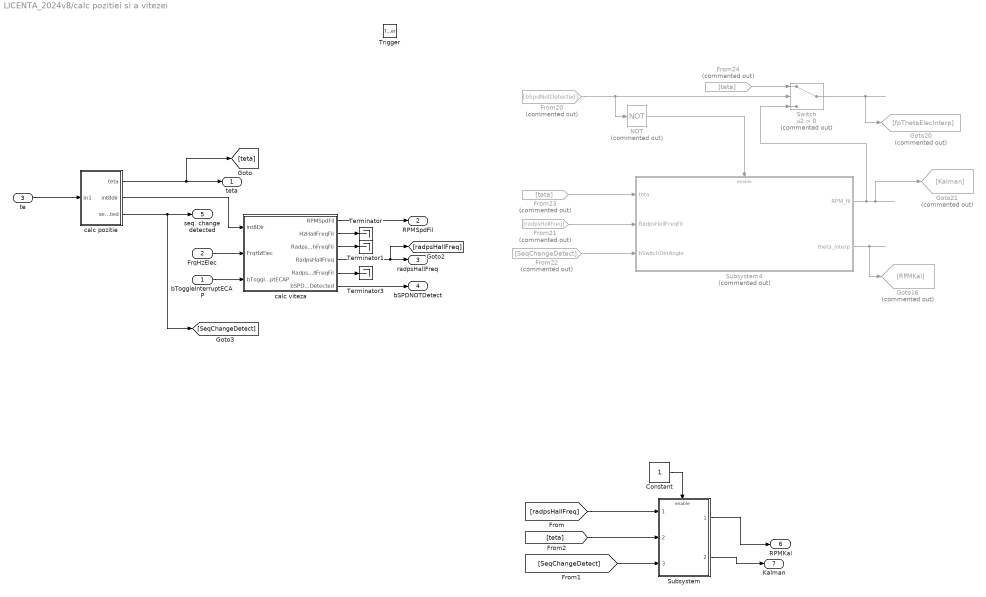
== system LICENTA_2024v8/calc pozitiei si a vitezei ==
  bToggleInterruptECAP : Inport
  FrqHzElec : Inport  Port=2
  te : Inport  Port=3
  Trigger : TriggerPort  TriggerType=function-call  VariantControl=(inherit)  PortDimensions=1
  Constant : Constant
  From20 : From  Commented=on  GotoTag=bSpdNotDetected
  From21 : From  Commented=on  GotoTag=radpsHallFreq
  From22 : From  Commented=on  GotoTag=SeqChangeDetect
  From23 : From  Commented=on  GotoTag=teta
  From24 : From  Commented=on  GotoTag=teta
  Goto16 : Goto  Commented=on  GotoTag=RPMKal
  Goto20 : Goto  Commented=on  GotoTag=fpThetaElecInterp
  Goto21 : Goto  Commented=on  GotoTag=Kalman
  NOT : Logic  Commented=on  Operator=NOT  IconShape=distinctive  AllPortsSameDT=off  OutDataTypeStr=boolean
  Subsystem : Subsystem
  Subsystem4 : Subsystem  Commented=on
  Switch : Switch  Commented=on  Criteria=u2 > Threshold
  Terminator : Terminator
  Terminator1 : Terminator
  Terminator3 : Terminator
  calc pozitie : Subsystem
  calc viteza : Subsystem
  teta : Outport  VectorParamsAs1DForOutWhenUnconnected=on
  RPMSpdFil : Outport  Port=2  VectorParamsAs1DForOutWhenUnconnected=on
  radpsHallFreq : Outport  Port=3  VectorParamsAs1DForOutWhenUnconnected=on
  "bSPDNOTDetect " : Outport  Port=4  VectorParamsAs1DForOutWhenUnconnected=on
  "seq. change detected " : Outport  Port=5  VectorParamsAs1DForOutWhenUnconnected=on
  RPMKal : Outport  Port=6  VectorParamsAs1DForOutWhenUnconnected=on
  Kalman : Outport  Port=7
  wires:
  bToggleInterruptECAP/1 -> calc viteza/3(bToggleInterruptECAP)
  calc viteza/1(RPMSpdFil) -> RPMSpdFil/1
  FrqHzElec/1 -> calc viteza/2(FrqHzElec)
  calc pozitie/2(int8dir) -> calc viteza/1(int8Dir)
  calc viteza/2(HzHallFreqFil) -> Terminator/1
  calc viteza/3(RadpsMechFreqFil) -> Terminator1/1
  calc viteza/5(RadpsHallFreqFil) -> Terminator3/1
  calc pozitie/1(teta) -> [teta], teta/1
  te/1 -> calc pozitie/1(In1)
  calc viteza/6(bSPDNOTDetected) -> "bSPDNOTDetect "/1
  calc viteza/4(RadpsHallFreq) -> [radpsHallFreq], radpsHallFreq/1
  calc pozitie/3("seq. change detected ") -> [SeqChangeDetect], "seq. change detected "/1
  From22/1 -> Subsystem4/3(bSwitchDetAngle)
  NOT/1 -> Subsystem4/Enable
  Subsystem4/2(theta_interp) -> Goto16/1
  From20/1 -> Switch/2, NOT/1
  Subsystem4/1(RPM_fil) -> Goto21/1, Switch/3
  From21/1 -> Subsystem4/2(RadpsHallFreqFil)
  Switch/1 -> Goto20/1
  From24/1 -> Switch/1
  From23/1 -> Subsystem4/1("teta ")
  Subsystem/1(RPMKal) -> RPMKal/1
  Subsystem/2(Kalman) -> Kalman/1
  Constant/1 -> Subsystem/Enable
  [radpsHallFreq] -> Subsystem/1(fPulsationElectricFiltered)
  [teta] -> Subsystem/2(fAngleElectricLowResolution)
  [SeqChangeDetect] -> Subsystem/3(bSwitchDetectedHall)

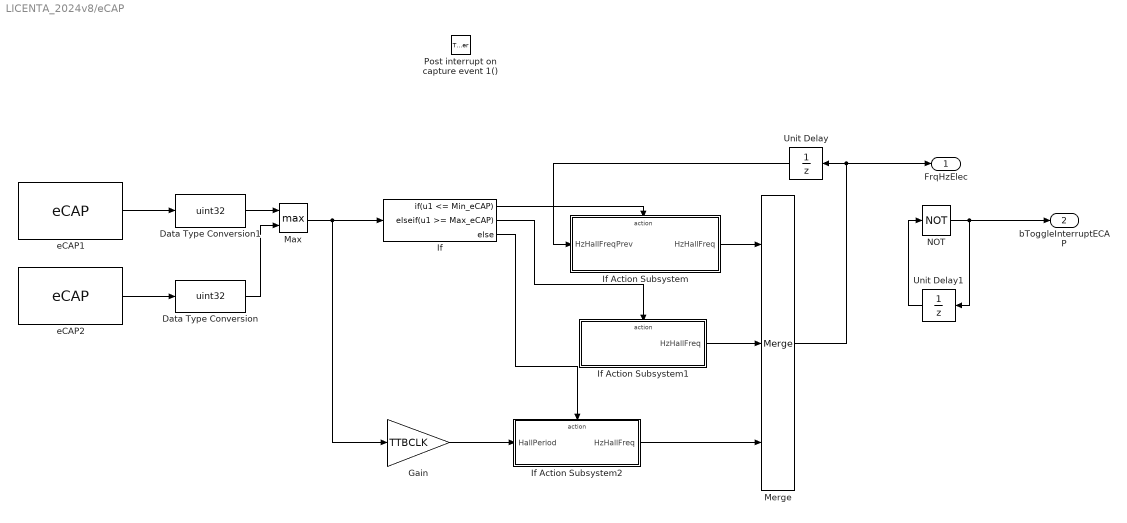
== system LICENTA_2024v8/eCAP ==
  Post interrupt on capture event 1() : TriggerPort  TriggerType=function-call  VariantControl=(inherit)  PortDimensions=1
  Data Type Conversion : DataTypeConversion  OutDataTypeStr=uint32
  Data Type Conversion1 : DataTypeConversion  OutDataTypeStr=uint32
  Gain : Gain  Gain=TTBCLK
  If : If  IfExpression=u1 <= Min_eCAP  ElseIfExpressions=u1 >= Max_eCAP
  If Action Subsystem : Subsystem  TreatAsAtomicUnit=on
  If Action Subsystem1 : Subsystem  TreatAsAtomicUnit=on
  If Action Subsystem2 : Subsystem  TreatAsAtomicUnit=on
  Max : MinMax  Function=max  Inputs=2
  Merge : Merge  Inputs=3
  NOT : Logic  Operator=NOT  IconShape=distinctive  AllPortsSameDT=off  OutDataTypeStr=boolean
  Unit Delay : UnitDelay  SampleTime=-1
  Unit Delay1 : UnitDelay  SampleTime=-1
  "eCAP1 " : c280xlib/eCAP  operatingMode=eCAP  selectCAPx=eCAP1  offsetValue=0  counterSynIn=off  enableCounter=off  syncOutput=Disabled  sampleTime=-1  eventPrescaler=0  selectMode=Continuous  enableOneShot=off  stopValue=Capture Event 1  resetEv1Ts=on  ev1Polarity=Rising Edge  resetEv2Ts=off  ev2Polarity=Rising Edge  resetEv3Ts=off  ev3Polarity=Rising Edge  resetEv4Ts=off  ev4Polarity=Rising Edge  tSCntrDataType=single  capEvFlag=off  capFlagDataType=uint16  overFlowFlag=off  overFlowFlagDataType=uint16  periodUnit=Seconds  periodSource=Specify via dialog  waveformPeriod=0.001  dutyUnit=Percentages  dutySource=Specify via dialog  dutyCycle=50  outputPolarity=Active High  enableCEVT1Int=on  enableCEVT2Int=off  enableCEVT3Int=off  enableCEVT4Int=off  enableCTROVFInt=off  enablePRDInt=off  enableCMPInt=off
      settings: SourceProductBaseCode=TIC2000
  "eCAP2 " : c280xlib/eCAP  operatingMode=eCAP  selectCAPx=eCAP2  offsetValue=0  counterSynIn=off  enableCounter=off  syncOutput=Disabled  sampleTime=-1  eventPrescaler=0  selectMode=Continuous  enableOneShot=off  stopValue=Capture Event 1  resetEv1Ts=on  ev1Polarity=Rising Edge  resetEv2Ts=off  ev2Polarity=Rising Edge  resetEv3Ts=off  ev3Polarity=Rising Edge  resetEv4Ts=off  ev4Polarity=Rising Edge  tSCntrDataType=single  capEvFlag=off  capFlagDataType=uint16  overFlowFlag=off  overFlowFlagDataType=uint16  periodUnit=Seconds  periodSource=Specify via dialog  waveformPeriod=0.001  dutyUnit=Percentages  dutySource=Specify via dialog  dutyCycle=50  outputPolarity=Active High  enableCEVT1Int=on  enableCEVT2Int=off  enableCEVT3Int=off  enableCEVT4Int=off  enableCTROVFInt=off  enablePRDInt=off  enableCMPInt=off
      settings: SourceProductBaseCode=TIC2000
  FrqHzElec : Outport
  bToggleInterruptECAP : Outport  Port=2
  wires:
  NOT/1 -> bToggleInterruptECAP/1, Unit Delay1/1
  Unit Delay1/1 -> NOT/1
  Unit Delay/1 -> If Action Subsystem/1(HzHallFreqPrev)
  Merge/1 -> FrqHzElec/1, Unit Delay/1
  Gain/1 -> If Action Subsystem2/1(HallPeriod)
  If Action Subsystem2/1(HzHallFreq) -> Merge/3
  If Action Subsystem1/1(HzHallFreq) -> Merge/2
  If Action Subsystem/1(HzHallFreq) -> Merge/1
  If/3 -> If Action Subsystem2/Action
  If/2 -> If Action Subsystem1/Action
  If/1 -> If Action Subsystem/Action
  Max/1 -> If/1, Gain/1
  Data Type Conversion1/1 -> Max/1
  Data Type Conversion/1 -> Max/2
  "eCAP1 "/1 -> Data Type Conversion1/1
  "eCAP2 "/1 -> Data Type Conversion/1

== system LICENTA_2024v8/PWM/Park Inverse ==
  d : Inport
  q : Inport  Port=2
  teta : Inport  Port=3
  Data Type Conversion : DataTypeConversion  OutDataTypeStr=fixdt(1,32,20)
  Data Type Conversion1 : DataTypeConversion  OutDataTypeStr=fixdt(1,32,20)
  IQN1 x IQN{1..4} (4 alike) : tiiqmathlib/IQN1 x IQN2  Q=20
      settings: SourceProductName=Embedded Coder Support Package for Texas Instruments C2000 Processors  SourceProductBaseCode=TIC2000
  Sum1 : Sum  Inputs=|++  OutDataTypeStr=Inherit: Same as first input
  Sum2 : Sum  Inputs=|+-  OutDataTypeStr=Inherit: Same as first input
  cos IQN : tiiqmathlib/Trig Fcn IQN  functionOption=_IQcos
      settings: SourceProductName=Embedded Coder Support Package for Texas Instruments C2000 Processors  SourceProductBaseCode=TIC2000
  sin IQN : tiiqmathlib/Trig Fcn IQN  functionOption=_IQsin
      settings: SourceProductName=Embedded Coder Support Package for Texas Instruments C2000 Processors  SourceProductBaseCode=TIC2000
  alpha : Outport
  beta : Outport  Port=2
  wires:
  teta/1 -> cos IQN/1, sin IQN/1
  Sum2/1 -> alpha/1
  d/1 -> Data Type Conversion/1
  sin IQN/1 -> IQN1 x IQN4/2, IQN1 x IQN1/2
  cos IQN/1 -> IQN1 x IQN3/2, IQN1 x IQN2/2
  q/1 -> Data Type Conversion1/1
  Sum1/1 -> beta/1
  IQN1 x IQN2/1 -> Sum2/1
  IQN1 x IQN1/1 -> Sum2/2
  IQN1 x IQN3/1 -> Sum1/1
  IQN1 x IQN4/1 -> Sum1/2
  Data Type Conversion/1 -> IQN1 x IQN4/1, IQN1 x IQN2/1
  Data Type Conversion1/1 -> IQN1 x IQN3/1, IQN1 x IQN1/1

== system LICENTA_2024v8/PWM/Subsystem ==
  Speed_ref : Inport
  KpPI : Inport  Port=2
  "KiPi " : Inport  Port=3
  RPMSpdFill : Inport  Port=4
  Ureg3 : Inport  Port=5
  Constant7 : Constant  Value=Ts
  Data Type Conversion : DataTypeConversion  OutDataTypeStr=single
  Product : Product
  Product1 : Product
  Product2 : Product
  Sum3 : Sum  Inputs=|++
  Sum4 : Sum  Inputs=|+-
  Sum5 : Sum  Inputs=|+-+
  Unit Delay : UnitDelay  SampleTime=-1
  Unit Delay1 : UnitDelay  SampleTime=-1
  "U PI " : Outport
  wires:
  "KiPi "/1 -> Product/1
  Ureg3/1 -> Unit Delay1/1
  KpPI/1 -> Sum3/2, Product2/1
  Sum5/1 -> Data Type Conversion/1
  Sum3/1 -> Product1/1
  Product2/1 -> Sum5/2
  Product1/1 -> Sum5/1
  Unit Delay/1 -> Product2/2
  Sum4/1 -> Unit Delay/1, Product1/2
  Unit Delay1/1 -> Sum5/3
  Constant7/1 -> Product/2
  Speed_ref/1 -> Sum4/1
  Product/1 -> Sum3/1
  RPMSpdFill/1 -> Sum4/2
  Data Type Conversion/1 -> "U PI "/1

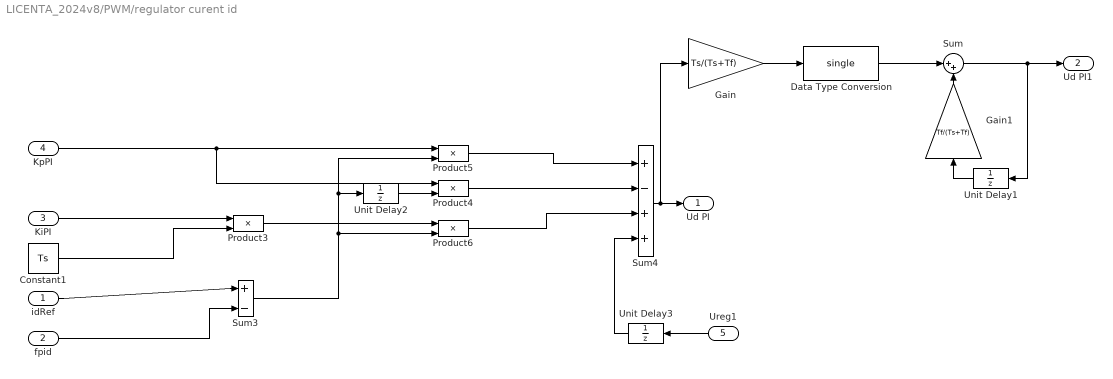
== system LICENTA_2024v8/PWM/regulator curent id ==
  idRef : Inport
  fpid : Inport  Port=2
  KiPI : Inport  Port=3
  KpPI : Inport  Port=4
  Ureg1 : Inport  Port=5
  Constant1 : Constant  Value=Ts  OutDataTypeStr=single  SampleTime=-1
  Data Type Conversion : DataTypeConversion  OutDataTypeStr=single
  Gain : Gain  Gain=Ts/(Ts+Tf)
  Gain1 : Gain  Gain=Tf/(Ts+Tf)
  Product{3..6} (4 alike) : Product
  Sum : Sum  Inputs=|++
  Sum3 : Sum  Inputs=|+-
  Sum4 : Sum  Inputs=+-++
  Unit Delay1 : UnitDelay  SampleTime=-1
  Unit Delay2 : UnitDelay  SampleTime=-1
  Unit Delay3 : UnitDelay  SampleTime=-1
  Ud PI : Outport
  Ud PI1 : Outport  Port=2
  wires:
  Product5/1 -> Sum4/1
  Product6/1 -> Sum4/3
  KpPI/1 -> Product4/1, Product5/1
  Ureg1/1 -> Unit Delay3/1
  Product4/1 -> Sum4/2
  Unit Delay3/1 -> Sum4/4
  Constant1/1 -> Product3/2
  idRef/1 -> Sum3/1
  KiPI/1 -> Product3/1
  fpid/1 -> Sum3/2
  Sum3/1 -> Product6/2, Product5/2, Unit Delay2/1
  Product3/1 -> Product6/1
  Gain1/1 -> Sum/2
  Gain/1 -> Data Type Conversion/1
  Unit Delay1/1 -> Gain1/1
  Sum/1 -> Ud PI1/1, Unit Delay1/1
  Sum4/1 -> Gain/1, Ud PI/1
  Unit Delay2/1 -> Product4/2
  Data Type Conversion/1 -> Sum/1

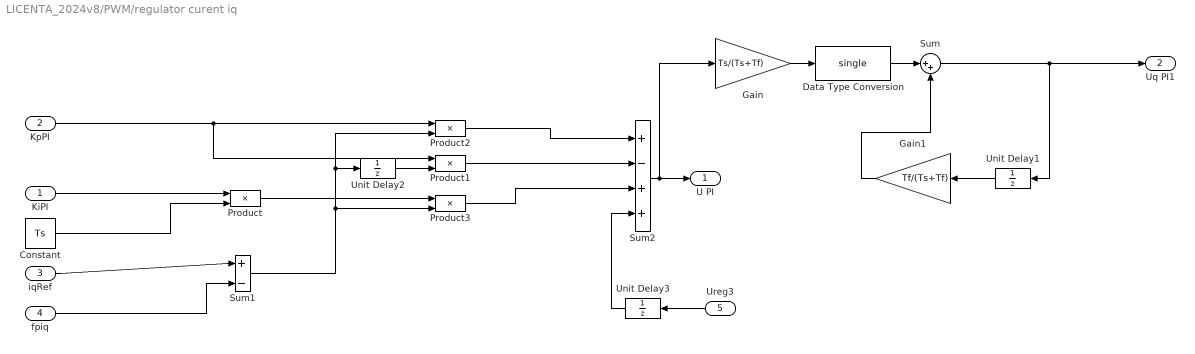
== system LICENTA_2024v8/PWM/regulator curent iq ==
  KiPI : Inport
  KpPI : Inport  Port=2
  iqRef : Inport  Port=3
  fpiq : Inport  Port=4
  Ureg3 : Inport  Port=5
  Constant : Constant  Value=Ts  OutDataTypeStr=single  SampleTime=-1
  Data Type Conversion : DataTypeConversion  OutDataTypeStr=single
  Gain : Gain  Gain=Ts/(Ts+Tf)
  Gain1 : Gain  Gain=Tf/(Ts+Tf)
  Product{,1..3} (4 alike) : Product
  Sum : Sum  Inputs=|++
  Sum1 : Sum  Inputs=|+-
  Sum2 : Sum  Inputs=+-++
  Unit Delay1 : UnitDelay  SampleTime=-1
  Unit Delay2 : UnitDelay  SampleTime=-1
  Unit Delay3 : UnitDelay  SampleTime=-1
  U PI : Outport
  Uq PI1 : Outport  Port=2
  wires:
  Sum2/1 -> Gain/1, U PI/1
  Sum1/1 -> Product3/2, Product2/2, Unit Delay2/1
  fpiq/1 -> Sum1/2
  iqRef/1 -> Sum1/1
  KiPI/1 -> Product/1
  Constant/1 -> Product/2
  Ureg3/1 -> Unit Delay3/1
  Unit Delay3/1 -> Sum2/4
  Product2/1 -> Sum2/1
  KpPI/1 -> Product1/1, Product2/1
  Product1/1 -> Sum2/2
  Product3/1 -> Sum2/3
  Product/1 -> Product3/1
  Gain/1 -> Data Type Conversion/1
  Sum/1 -> Uq PI1/1, Unit Delay1/1
  Unit Delay1/1 -> Gain1/1
  Gain1/1 -> Sum/2
  Unit Delay2/1 -> Product1/2
  Data Type Conversion/1 -> Sum/1

== system LICENTA_2024v8/Subsystem/3value average ==
  in : Inport
  Gain : Gain  Gain=1/3  OutDataTypeStr=fixdt(1,32,16)
  Sum : Sum  Inputs=3
  Unit Delay : UnitDelay  SampleTime=-1
  Unit Delay1 : UnitDelay  SampleTime=-1
  out : Outport
  wires:
  Sum/1 -> Gain/1
  Gain/1 -> out/1
  in/1 -> Unit Delay1/1, Sum/1
  Unit Delay1/1 -> Sum/2, Unit Delay/1
  Unit Delay/1 -> Sum/3

== system LICENTA_2024v8/Subsystem/3value average1 ==
  in : Inport
  Gain : Gain  Gain=1/3  OutDataTypeStr=fixdt(1,32,16)
  Sum : Sum  Inputs=3
  Unit Delay : UnitDelay  SampleTime=-1
  Unit Delay1 : UnitDelay  SampleTime=-1
  out : Outport
  wires:
  Unit Delay/1 -> Sum/3
  Unit Delay1/1 -> Unit Delay/1, Sum/2
  in/1 -> Sum/1, Unit Delay1/1
  Gain/1 -> out/1
  Sum/1 -> Gain/1

== system LICENTA_2024v8/Subsystem/3value average2 ==
  in : Inport
  Gain : Gain  Gain=1/3  OutDataTypeStr=fixdt(1,32,16)
  Sum : Sum  Inputs=3
  Unit Delay : UnitDelay  SampleTime=-1
  Unit Delay1 : UnitDelay  SampleTime=-1
  out : Outport
  wires:
  Unit Delay/1 -> Sum/3
  Unit Delay1/1 -> Unit Delay/1, Sum/2
  in/1 -> Sum/1, Unit Delay1/1
  Gain/1 -> out/1
  Sum/1 -> Gain/1

== system LICENTA_2024v8/Subsystem/3value average3 ==
  in : Inport
  Gain : Gain  Gain=1/3  OutDataTypeStr=fixdt(1,32,16)
  Sum : Sum  Inputs=3
  Unit Delay : UnitDelay  SampleTime=-1
  Unit Delay1 : UnitDelay  SampleTime=-1
  out : Outport
  wires:
  Sum/1 -> Gain/1
  Gain/1 -> out/1
  in/1 -> Unit Delay1/1, Sum/1
  Unit Delay1/1 -> Sum/2, Unit Delay/1
  Unit Delay/1 -> Sum/3

== system LICENTA_2024v8/Subsystem/3value average4 ==
  in : Inport
  Gain : Gain  Gain=1/3  OutDataTypeStr=fixdt(1,32,16)
  Sum : Sum  Inputs=3
  Unit Delay : UnitDelay  SampleTime=-1
  Unit Delay1 : UnitDelay  SampleTime=-1
  out : Outport
  wires:
  Sum/1 -> Gain/1
  Gain/1 -> out/1
  in/1 -> Unit Delay1/1, Sum/1
  Unit Delay1/1 -> Sum/2, Unit Delay/1
  Unit Delay/1 -> Sum/3

== system LICENTA_2024v8/Subsystem/transf clarke ==
  fISENA : Inport
  fISENB : Inport  Port=2
  fISENC : Inport  Port=3
  Float to IQN2 : tiiqmathlib/Float to IQN  Q_value=18
      settings: SourceProductBaseCode=TIC2000
  Float to IQN3 : tiiqmathlib/Float to IQN  Q_value=18
      settings: SourceProductBaseCode=TIC2000
  Gain : Gain  Gain=2/3  OutDataTypeStr=fixdt(1,32,16)
  Gain1 : Gain  Gain=-1/3  OutDataTypeStr=fixdt(1,32,16)
  Gain2 : Gain  Gain=-1/3  OutDataTypeStr=fixdt(1,32,16)
  Gain3 : Gain  Gain=sqrt(3)/3  OutDataTypeStr=fixdt(1,32,16)
  Gain4 : Gain  Gain=-sqrt(3)/3  OutDataTypeStr=fixdt(1,32,16)
  Sum : Sum  Inputs=|+++  OutDataTypeStr=single
  Sum1 : Sum  Inputs=|++  AccumDataTypeStr=single  OutDataTypeStr=single
  fpIalfa : Outport
  fpIbeta : Outport  Port=2
  wires:
  Gain3/1 -> Sum1/1
  Gain4/1 -> Sum1/2
  Gain2/1 -> Sum/3
  Gain1/1 -> Sum/2
  fISENC/1 -> Gain4/1, Gain2/1
  Gain/1 -> Sum/1
  fISENB/1 -> Gain1/1, Gain3/1
  fISENA/1 -> Gain/1
  Float to IQN2/1 -> fpIalfa/1
  Float to IQN3/1 -> fpIbeta/1
  Sum1/1 -> Float to IQN3/1
  Sum/1 -> Float to IQN2/1

== system LICENTA_2024v8/Subsystem/transf park ==
  alpha : Inport
  beta : Inport  Port=2
  "teta " : Inport  Port=3
  IQN1 x IQN{,1..3} (4 alike) : tiiqmathlib/IQN1 x IQN2  Q=20
      settings: SourceProductName=Embedded Coder Support Package for Texas Instruments C2000 Processors  SourceProductBaseCode=TIC2000
  Sum3 : Sum  Inputs=|++
  Sum4 : Sum  Inputs=|-+
  cos : tiiqmathlib/Trig Fcn IQN  functionOption=_IQcos
      settings: SourceProductName=Embedded Coder Support Package for Texas Instruments C2000 Processors  SourceProductBaseCode=TIC2000
  sin : tiiqmathlib/Trig Fcn IQN  functionOption=_IQsin
      settings: SourceProductName=Embedded Coder Support Package for Texas Instruments C2000 Processors  SourceProductBaseCode=TIC2000
  d : Outport
  q : Outport  Port=2
  wires:
  Sum3/1 -> d/1
  Sum4/1 -> q/1
  "teta "/1 -> sin/1, cos/1
  IQN1 x IQN1/1 -> Sum3/1  "beta*sin(theta)"
  IQN1 x IQN2/1 -> Sum3/2  "alpha*cos(theta)"
  IQN1 x IQN3/1 -> Sum4/2  "beta*cos(theta)"
  IQN1 x IQN/1 -> Sum4/1  "alpha*sin(theta)"
  cos/1 -> IQN1 x IQN3/1, IQN1 x IQN2/2
  sin/1 -> IQN1 x IQN1/1, IQN1 x IQN/2
  alpha/1 -> IQN1 x IQN2/1, IQN1 x IQN/1
  beta/1 -> IQN1 x IQN1/2, IQN1 x IQN3/2
